simulink model "RL_Traction_motor_torch"  (R2022a)
settings: Solver=FixedStepAuto  StartTime=0.0  StopTime=0.25  FixedStep=5E-6  RelTol=1e-3
model workspace (MAT data in the model file):
  Cdc = 0.001
  Jm = 0.1234
  Ki_id = 710.3004
  Ki_iq = 1061.5
  Ki_omega = 500
  Kp_id = 0.8779
  Kp_iq = 1.0744
  Kp_omega = 20
  L0 = 0.00012184
  Ld = 0.00024368
  LdMatrix = [0.000182 0.00018 0.000178 0.000177 0.000176 0.00017475 0.0001735 0.00017247 0.00017132 0.00016571 0.00016537 0.00016571 ... (735 elements, 21x35)]
  Lq = 0.00029758
  LqMatrix = [0.000217 0.000217 0.000217 0.000217 0.000217 0.0002145 0.000212 0.0002115 0.00021022 0.0002079 0.00020461 0.0002079 ... (735 elements, 21x35)]
  PmMatrix = [0.0363 0.0363 0.0363 0.0363 0.0363 0.0363 0.0363 0.0363 0.0363 0.0363 0.0363 0.0363 ... (735 elements, 21x35)]
  Pmax = 35000
  Rs = 0.010087
  Tmax = 200
  Ts = 5e-06
  Tsc = 0.0001
  V1 = 290
  Vnom = 325
  fsw = 10000
  idVec = [-250 -225 -200 -175 -150 -125 -100 -75 -50 -25 0 25 ... (21 elements, 1x21)]
  iqVec = [-425 -400 -375 -350 -325 -300 -275 -250 -225 -200 -175 -150 ... (35 elements, 1x35)]
  p = 8
  psim = 0.044
undefined symbols (not defined in the file or in its folder): ee_sli_rtmsupport, gcbh, idMatrix, Imax, iqMatrix, rpmVec, TqVec, VdcVec
libraries: fl_lib x19, nesl_utility x13, eeGeneralControl x9, ee_lib x7, slpidlib x5, simulink x3, eeTransforms x2, eeDqVoltageLimiter x1, eePwmGeneratorTwoLevel x1, eeResolverToDigitalConverter x1
(part 3 of 3)

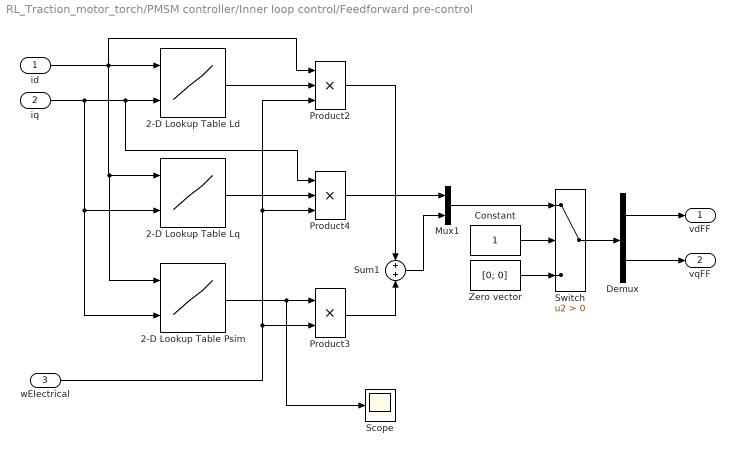
== system RL_Traction_motor_torch/PMSM controller/Inner loop control/Feedforward pre-control ==
  id : Inport
  iq : Inport  Port=2
  wElectrical : Inport  Port=3
  2-D Lookup Table Ld : Lookup_n-D  BreakpointsForDimension1=idVec  BreakpointsForDimension2=iqVec  Table=LdMatrix  ExtrapMethod=Clip  UseLastTableValue=on  InternalRulePriority=Speed  RndMeth=Simplest
      settings: InputPortMap=u0,u1
  2-D Lookup Table Lq : Lookup_n-D  BreakpointsForDimension1=idVec  BreakpointsForDimension2=iqVec  Table=LqMatrix  ExtrapMethod=Clip  InternalRulePriority=Speed  RndMeth=Simplest
      settings: InputPortMap=u0,u1
  2-D Lookup Table Psim : Lookup_n-D  BreakpointsForDimension1=idVec  BreakpointsForDimension2=iqVec  Table=PmMatrix  ExtrapMethod=Clip  InternalRulePriority=Speed  RndMeth=Simplest
      settings: InputPortMap=u0,u1
  Constant : Constant  SampleTime=Tsc
  Demux : Demux  Outputs=2
  Mux1 : Mux  Inputs=2
  Product2 : Product  Inputs=3
  Product3 : Product
  Product4 : Product  Inputs=3
  Scope : Scope
  Sum1 : Sum
  Switch : Switch  Criteria=u2 > Threshold  SaturateOnIntegerOverflow=off  InputSameDT=off
  Zero vector : Constant  Value=[0; 0]  SampleTime=Tsc
  vdFF : Outport  VectorParamsAs1DForOutWhenUnconnected=off
  vqFF : Outport  Port=2  VectorParamsAs1DForOutWhenUnconnected=off
  wires:
  Product3/1 -> Sum1/2
  2-D Lookup Table Lq/1 -> Product4/2
  Constant/1 -> Switch/2
  Switch/1 -> Demux/1
  Demux/1 -> vdFF/1
  Demux/2 -> vqFF/1
  2-D Lookup Table Psim/1 -> Scope/1, Product3/1
  Zero vector/1 -> Switch/3
  Sum1/1 -> Mux1/2
  2-D Lookup Table Ld/1 -> Product2/2
  iq/1 -> Product4/1, 2-D Lookup Table Ld/2, 2-D Lookup Table Lq/2, 2-D Lookup Table Psim/2
  id/1 -> Product2/1, 2-D Lookup Table Psim/1, 2-D Lookup Table Lq/1, 2-D Lookup Table Ld/1
  Product4/1 -> Mux1/1
  Mux1/1 -> Switch/1
  wElectrical/1 -> Product3/2, Product4/3, Product2/3
  Product2/1 -> Sum1/1

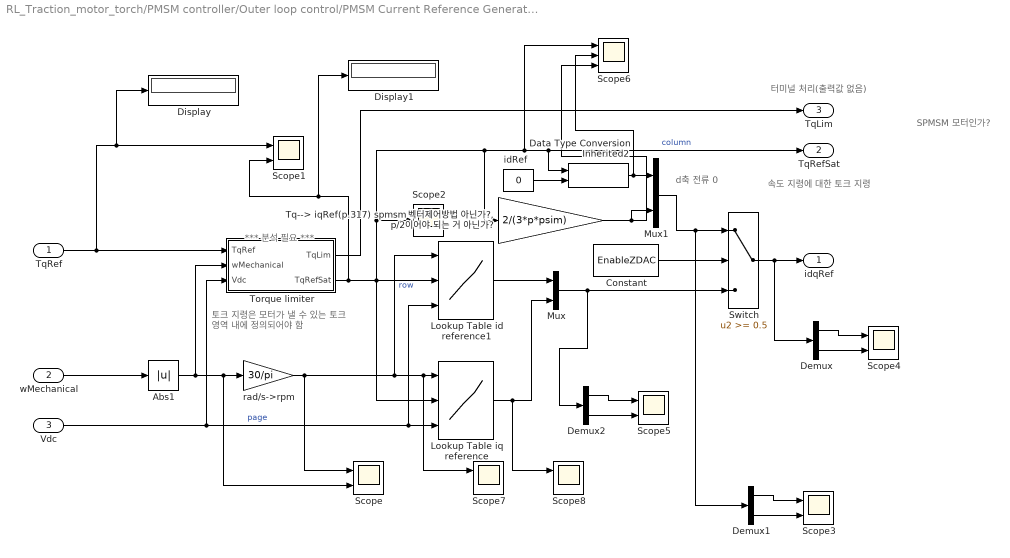
== system RL_Traction_motor_torch/PMSM controller/Outer loop control/PMSM Current Reference Generator ==
  note: SPMSM 모터인가?
  note: d축 전류 0
  note: *** 분석 필요 ***
  note: 토크 지령은 모터가 낼 수 있는
      | 토크 영역 내에 정의되어야 함
  note: 속도 지령에 대한 토크 지령
  note: 터미널 처리(출력값 없음)
  TqRef : Inport  SampleTime=Ts
  wMechanical : Inport  Port=2  SampleTime=Ts
  Vdc : Inport  Port=3  SampleTime=Ts
  Abs1 : Abs  SaturateOnIntegerOverflow=off
  Constant : Constant  Value=EnableZDAC  VectorParams1D=off  SampleTime=Ts
  Data Type Conversion Inherited2 : simulink/Signal Attributes/Data Type Conversion Inherited  ConvertRealWorld=Real World Value  DoSatur=off
      settings: SourceProductBaseCode=SL
  Demux : Demux  Outputs=2
  Demux1 : Demux  Outputs=2
  Demux2 : Demux  Outputs=2
  Display : Display
  Display1 : Display
  Lookup Table id reference1 : Lookup_n-D  NumberOfTableDimensions=3  BreakpointsForDimension1=rpmVec  BreakpointsForDimension2=TqVec  BreakpointsForDimension3=VdcVec  Table=idMatrix
      settings: InputPortMap=u0,u1,u2
  Lookup Table iq reference : Lookup_n-D  NumberOfTableDimensions=3  BreakpointsForDimension1=rpmVec  BreakpointsForDimension2=TqVec  BreakpointsForDimension3=VdcVec  Table=iqMatrix
      settings: InputPortMap=u0,u1,u2
  Mux : Mux  Inputs=2
  Mux1 : Mux  Inputs=2
  Scope{,1,3..5,7..8} (7 alike) : Scope  NumInputPorts=2
  Scope2 : Scope
  Scope6 : Scope  NumInputPorts=3
  Switch : Switch  Threshold=0.5  SaturateOnIntegerOverflow=off  InputSameDT=off
  Torque limiter : Subsystem
  "Tq--> iqRef(p.317) spmsm 벡터제어방법 아닌가?, p/2이어야 되는 거 아닌가? " : Gain  Gain=2/(3*p*psim)
  idRef : Constant  Value=0  SampleTime=Ts
  rad/s->rpm : Gain  Gain=30/pi
  idqRef : Outport  VectorParamsAs1DForOutWhenUnconnected=off
  TqRefSat : Outport  Port=2  VectorParamsAs1DForOutWhenUnconnected=off
  TqLim : Outport  Port=3  VectorParamsAs1DForOutWhenUnconnected=off
  wires:
  idRef/1 -> Data Type Conversion Inherited2/2
  Lookup Table id reference1/1 -> Mux/1
  Lookup Table iq reference/1 -> Scope8/1, Mux/2
  Torque limiter/2(TqRefSat) -> Display1/1, Scope1/2, Lookup Table id reference1/2, Lookup Table iq reference/2, "Tq--> iqRef(p.317) spmsm 벡터제어방법 아닌가?, p/2이어야 되는 거 아닌가? "/1, Scope6/1, TqRefSat/1, Data Type Conversion Inherited2/1, Scope2/1  "column"
  Torque limiter/1(TqLim) -> TqLim/1
  rad/s->rpm/1 -> Scope/1, Lookup Table id reference1/1, Scope7/1, Lookup Table iq reference/1  "row"
  Abs1/1 -> Torque limiter/2(wMechanical), Scope/2, rad/s->rpm/1
  Mux/1 -> Demux2/1, Switch/3
  Switch/1 -> Demux/1, idqRef/1
  Data Type Conversion Inherited2/1 -> Mux1/1, Scope6/2
  "Tq--> iqRef(p.317) spmsm 벡터제어방법 아닌가?, p/2이어야 되는 거 아닌가? "/1 -> Scope6/3, Mux1/2
  TqRef/1 -> Display/1, Scope1/1, Torque limiter/1(TqRef)
  wMechanical/1 -> Abs1/1
  Vdc/1 -> Lookup Table id reference1/3, Lookup Table iq reference/3, Torque limiter/3(Vdc)  "page"
  Constant/1 -> Switch/2
  Demux/2 -> Scope4/2
  Demux/1 -> Scope4/1
  Demux1/2 -> Scope3/2
  Demux1/1 -> Scope3/1
  Mux1/1 -> Demux1/1, Switch/1
  Demux2/2 -> Scope5/2
  Demux2/1 -> Scope5/1

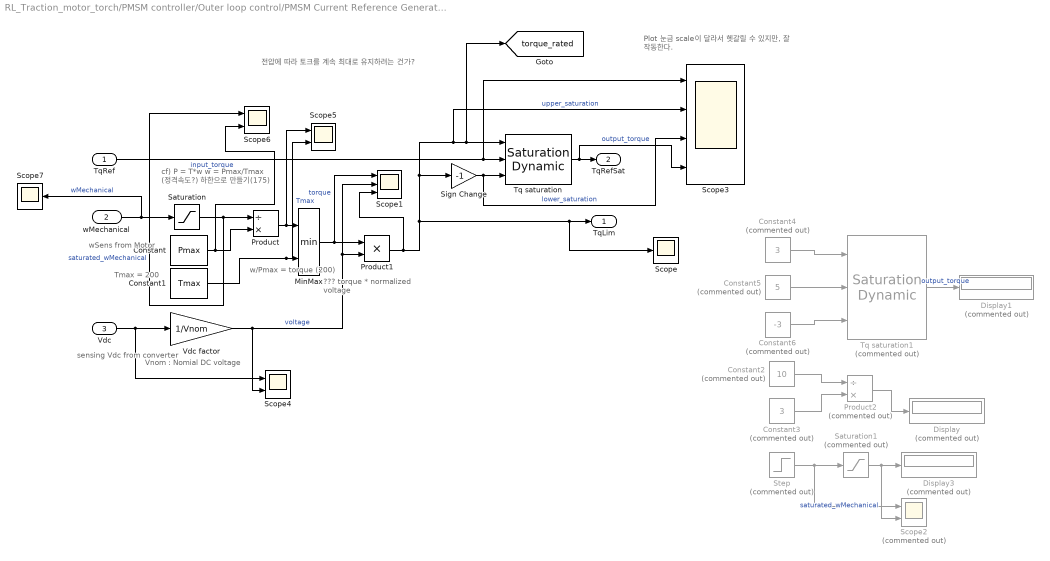
== system RL_Traction_motor_torch/PMSM controller/Outer loop control/PMSM Current Reference Generator/Torque limiter ==
  note: Plot 눈금 scale이 달라서 헷갈릴 수 있지만,
      | 잘 작동한다.
  note: Tmax = 200
  note: 전압에 따라 토크를 계속 최대로 유지하려는 건가?
  note: wSens
      | from Motor
  note: ???
      | torque * normalized voltage
  note: w/Pmax
      | = torque
      | (200)
  note: sensing Vdc
      | from converter
  note: Vnom : Nomial DC voltage
  note: cf) P = T*w
      | w = Pmax/Tmax (정격속도?)
      | 하한으로 만들기(175)
  TqRef : Inport
  wMechanical : Inport  Port=2
  Vdc : Inport  Port=3
  Constant : Constant  Value=Pmax  SampleTime=Ts
  Constant1 : Constant  Value=Tmax  SampleTime=Ts
  Constant2 : Constant  Commented=on  Value=10
  Constant3 : Constant  Commented=on  Value=3
  Constant4 : Constant  Commented=on  Value=3
  Constant5 : Constant  Commented=on  Value=5
  Constant6 : Constant  Commented=on  Value=-3
  Display : Display  Commented=on
  Display1 : Display  Commented=on
  Display3 : Display  Commented=on
  MinMax : MinMax  Inputs=2  OutDataTypeStr=Inherit: Same as first input
  Product : Product  Inputs=/*  OutDataTypeStr=Inherit: Same as first input
  Product1 : Product
  Product2 : Product  Commented=on  Inputs=/*
  Saturation : Saturate  UpperLimit=inf  LowerLimit=Pmax/Tmax
  Saturation1 : Saturate  Commented=on  UpperLimit=inf  LowerLimit=100
  Scope : Scope
  Scope1 : Scope  NumInputPorts=3
  Scope2 : Scope  Commented=on  NumInputPorts=2
  Scope3 : Scope  NumInputPorts=4
  Scope4 : Scope  NumInputPorts=2
  Scope5 : Scope  NumInputPorts=2
  Scope6 : Scope  NumInputPorts=2
  Scope7 : Scope
  Sign Change : Gain  Gain=-1
  Step : Step  Commented=on  Time=0  After=1000  SampleTime=0
  Tq saturation : simulink/Discontinuities/Saturation Dynamic  OutMin=[]  OutMax=[]  OutDataTypeStr=Inherit: Same as second input  OutDataType=fixdt(1, 16)  OutScaling=2^-10  DoSatur=off
  Tq saturation1 : simulink/Discontinuities/Saturation Dynamic  Commented=on  OutMin=[]  OutMax=[]  OutDataTypeStr=Inherit: Same as second input  OutDataType=fixdt(1, 16)  OutScaling=2^-10  DoSatur=off
  Vdc factor : Gain  Gain=1/Vnom
  TqLim : Outport  VectorParamsAs1DForOutWhenUnconnected=off
  TqRefSat : Outport  Port=2  VectorParamsAs1DForOutWhenUnconnected=off
  tag scope: torque_rated=global
  wires:
  Saturation/1 -> Scope6/1, Product/1  "saturated_wMechanical"
  Tq saturation/1 -> Scope3/4, TqRefSat/1  "output_torque"
  Product1/1 -> Scope1/3, Scope3/2, [torque_rated], Tq saturation/1, Sign Change/1, Scope/1, TqLim/1  "upper_saturation"
  TqRef/1 -> Scope3/1, Tq saturation/2  "input_torque"
  Constant1/1 -> Scope5/2, MinMax/2  "Tmax"
  wMechanical/1 -> Scope7/1, Saturation/1  "wMechanical"
  Product/1 -> Scope5/1, MinMax/1
  Sign Change/1 -> Scope3/3, Tq saturation/3  "lower_saturation"
  MinMax/1 -> Scope1/1, Product1/1  "torque"
  Vdc factor/1 -> Scope1/2, Product1/2, Scope4/2  "voltage"
  Constant/1 -> Scope6/2, Product/2
  Step/1 -> Scope2/1, Saturation1/1
  Saturation1/1 -> Scope2/2, Display3/1  "saturated_wMechanical"
  Vdc/1 -> Scope4/1, Vdc factor/1
  Constant2/1 -> Product2/1
  Constant3/1 -> Product2/2
  Product2/1 -> Display/1
  Constant4/1 -> Tq saturation1/1
  Constant5/1 -> Tq saturation1/2
  Constant6/1 -> Tq saturation1/3
  Tq saturation1/1 -> Display1/1  "output_torque"

== matlab function RL_Traction_motor_torch/Subsystem/r(error_norm, constraints) ==
  data: u input; y output
function y = fcn(u)

y = u;

== matlab function RL_Traction_motor_torch/Subsystem/r(error_norm, constraints)1 ==
  data: u input; y output
function y = fcn(u)

y = u;
